simulink model "Marine_LocoMotive_UAV"  (R2018a)
settings: Solver=ode4  StartTime=0.0  StopTime=60  FixedStep=T  RelTol=1e-3
values from neighbouring files (symbols this model uses):
  a_11 = 0.05*m_b    (= 0.625)    [Marine_LocoMotive_UAV_parameters.m]
  a_33 = m_b    (= 12.5)    [Marine_LocoMotive_UAV_parameters.m]
  A_w = 1*1.5/2    (= 0.75)    [Marine_LocoMotive_UAV_parameters.m]
  A_w2 = 1*0.27/2    (= 0.135)    [Marine_LocoMotive_UAV_parameters.m]
  alpha_bar = pi/4    (= 0.785398163397)    [Marine_LocoMotive_UAV_parameters.m]
  Am = sysd.denominator{1}    [Marine_LocoMotive_UAV_parameters.m]
  Am1_LPF = sysd.denominator{1}    [Marine_LocoMotive_UAV_parameters.m]
  Am2_LPF = sysd.denominator{1}    [Marine_LocoMotive_UAV_parameters.m]
  AmAlpha_LPF = sysd.denominator{1}    [Marine_LocoMotive_UAV_parameters.m]
  AmV_LPF = sysd.denominator{1}    [Marine_LocoMotive_UAV_parameters.m]
  AmZ_LPF = sysd.denominator{1}    [Marine_LocoMotive_UAV_parameters.m]
  b_11 = 0    [Marine_LocoMotive_UAV_parameters.m]
  b_33 = 2*m_b*omega_h    (= 27.5578302946)    [Marine_LocoMotive_UAV_parameters.m]
  Bm = sysd.numerator{1}    [Marine_LocoMotive_UAV_parameters.m]
  Bm1_LPF = sysd.numerator{1}    [Marine_LocoMotive_UAV_parameters.m]
  Bm2_LPF = sysd.numerator{1}    [Marine_LocoMotive_UAV_parameters.m]
  BmAlpha_LPF = sysd.numerator{1}    [Marine_LocoMotive_UAV_parameters.m]
  BmV_LPF = sysd.numerator{1}    [Marine_LocoMotive_UAV_parameters.m]
  BmZ_LPF = sysd.numerator{1}    [Marine_LocoMotive_UAV_parameters.m]
  C_S = [5;9]*10^-3    [Marine_LocoMotive_UAV_parameters.m]
  D_x = b_11 + D_s(1)    [Marine_LocoMotive_UAV_parameters.m]
  D_z = b_33 + D_s(2)    [Marine_LocoMotive_UAV_parameters.m]
  dc_M_p = 6.7    [Marine_LocoMotive_UAV_parameters.m]
  Delta_h = (A_im/A_b-0.5)*h_b    (= -0.0625)    [Marine_LocoMotive_UAV_parameters.m]
  epsilon_1 = 5    [Marine_LocoMotive_UAV_parameters.m]
  epsilon_w = 0    [Marine_LocoMotive_UAV_parameters.m]
  epsilon_w2 = pi    (= 3.14159265359)    [Marine_LocoMotive_UAV_parameters.m]
  g = 9.81    [Marine_LocoMotive_UAV_parameters.m]
  gamma_d_p = 2*0.3/0.03*2*0.2*12/4    (= 24)    [Marine_LocoMotive_UAV_parameters.m]
  H = 10    [Marine_LocoMotive_UAV_parameters.m]
  h_b = 0.25    [Marine_LocoMotive_UAV_parameters.m]
  J_a = m_u*Lc_0^2 + (m_u*(Lc_0/2)^2+m_u*Lc_0/12)    (= 111.3)    [Marine_LocoMotive_UAV_parameters.m]
  J_b = m_b*h_b*l_b/12    (= 0.208333333333)    [Marine_LocoMotive_UAV_parameters.m]
  J_u = 0.03    [Marine_LocoMotive_UAV_parameters.m]
  K = 20    [Marine_LocoMotive_UAV_parameters.m]
  k3 = 4.5    [Marine_LocoMotive_UAV_parameters.m]
  k4 = 2    [Marine_LocoMotive_UAV_parameters.m]
  k_w = omega_w^2/g    (= 0.123862835563)    [Marine_LocoMotive_UAV_parameters.m]
  k_w2 = omega_w2^2/g    (= 0.447144836384)    [Marine_LocoMotive_UAV_parameters.m]
  kd_a = 7    [Marine_LocoMotive_UAV_parameters.m]
  kd_t = 6    [Marine_LocoMotive_UAV_parameters.m]
  kd_T = 0.3    [Marine_LocoMotive_UAV_parameters.m]
  kd_x = 5    [Marine_LocoMotive_UAV_parameters.m]
  kd_z = 2    [Marine_LocoMotive_UAV_parameters.m]
  ki_a = 2    [Marine_LocoMotive_UAV_parameters.m]
  ki_T = 0.8    [Marine_LocoMotive_UAV_parameters.m]
  ki_x = 1.2    [Marine_LocoMotive_UAV_parameters.m]
  ki_z = 1    [Marine_LocoMotive_UAV_parameters.m]
  kp_a = 7    [Marine_LocoMotive_UAV_parameters.m]
  kp_t = 10    [Marine_LocoMotive_UAV_parameters.m]
  kp_T = 5    [Marine_LocoMotive_UAV_parameters.m]
  kp_x = 7    [Marine_LocoMotive_UAV_parameters.m]
  kp_z = 3    [Marine_LocoMotive_UAV_parameters.m]
  L = 0.2    [Marine_LocoMotive_UAV_parameters.m]
  l_b = 0.8    [Marine_LocoMotive_UAV_parameters.m]
  Lc_0 = 7    [Marine_LocoMotive_UAV_parameters.m]
  LIMIT_CMD_PITCH = 45*pi/180    (= 0.785398163397)    [Marine_LocoMotive_UAV_parameters.m]
  LIMIT_uCMD_HEIGHT = 3.5*K    (= 70)    [Marine_LocoMotive_UAV_parameters.m]
  M_a = m_u*Lc_0 + m_c*Lc_0    (= 16.1)    [Marine_LocoMotive_UAV_parameters.m]
  m_b = rho_w*Vol_b/4    (= 12.5)    [Marine_LocoMotive_UAV_parameters.m]
  m_c = 0.5    [Marine_LocoMotive_UAV_parameters.m]
  m_u = 1.8    [Marine_LocoMotive_UAV_parameters.m]
  nu_w = 1.787*10^-6    (= 1.787e-06)    [Marine_LocoMotive_UAV_parameters.m]
  omega_w = 2*pi/T_w    (= 1.10231321179)    [Marine_LocoMotive_UAV_parameters.m]
  omega_w2 = 2*pi/T_w2    (= 2.09439510239)    [Marine_LocoMotive_UAV_parameters.m]
  rho_w = 1000    [Marine_LocoMotive_UAV_parameters.m]
  T = 1/100    (= 0.01)    [Marine_LocoMotive_UAV_parameters.m]
  Theta0 = atan2(V_bar*D_x*cos(alpha_bar_0),V_bar*D_x*sin(alpha_bar_0)+m_u*g*cos(alpha_bar_0))    [Marine_LocoMotive_UAV_parameters.m]
  u_s = w_dir*A_w^2*omega_w*k_w*exp(2*k_w*(-Delta_h/2))    [Marine_LocoMotive_UAV_parameters.m]
  u_s2 = w_dir2*A_w2^2*omega_w2*k_w2*exp(2*k_w2*(-Delta_h/2))    [Marine_LocoMotive_UAV_parameters.m]
  u_t = 0*0.2*1    (= 0)    [Marine_LocoMotive_UAV_parameters.m]
  u_w = 0*0.2    (= 0)    [Marine_LocoMotive_UAV_parameters.m]
  V0_b = [u_t+u_w+u_s+u_s2+v_x_w, v_z_w]    [Marine_LocoMotive_UAV_parameters.m]
  V_bar = 5    [Marine_LocoMotive_UAV_parameters.m]
  Vol_b = A_b*l_b    (= 0.05)    [Marine_LocoMotive_UAV_parameters.m]
  w_dir = 1    [Marine_LocoMotive_UAV_parameters.m]
  w_dir2 = 1    [Marine_LocoMotive_UAV_parameters.m]
  X0_b = [0,H+Zeta_0-Delta_h]    [Marine_LocoMotive_UAV_parameters.m]
  zu_bar = X0_b(2) + Lc_0*sin(alpha_bar_0)    [Marine_LocoMotive_UAV_parameters.m]
undefined symbols (not defined in the file or in its folder): DiscIntNeverNeededParam, k_Da, k_Pa, R_b, Zg
libraries: simulink x30, simulink_extras x3
(part 2 of 3)

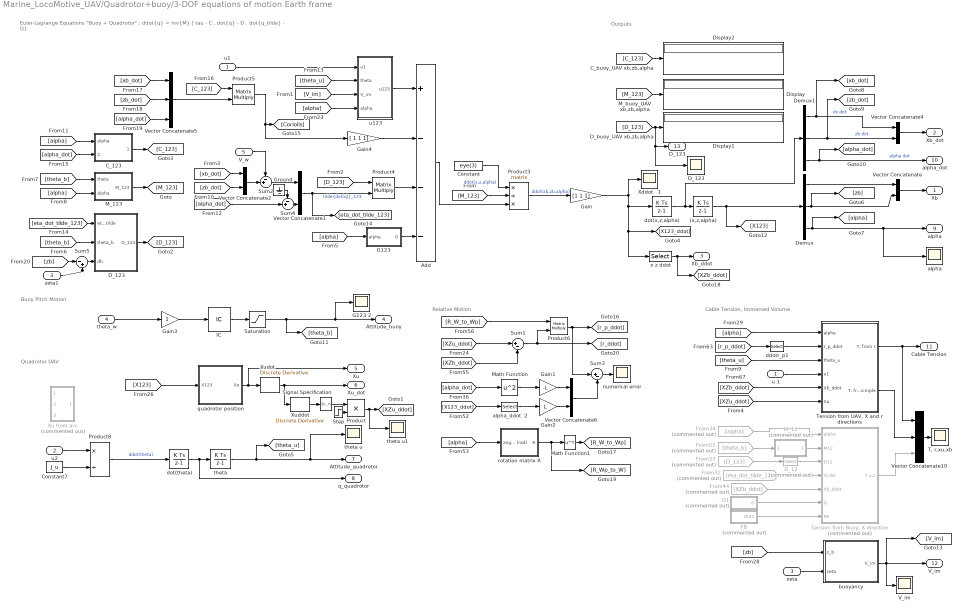
== system Marine_LocoMotive_UAV/Quadrotor+buoy/3-DOF equations of motion Earth frame ==
  note: Relative Motion
  note: Outputs
  note: Buoy Pitch Motion
  note: Cable Tension, Immersed Volume
  note: Quadrotor UAV
  note: Euler-Lagrange Equations "Buoy + Quadrotor" : ddot{q} = inv{M} [ tau - C . dot{q} - D . dot{q_tilde} - G]
  u1 : Inport
  u2 : Inport  Port=2
  zeta : Inport  Port=3
  theta_w : Inport  Port=4
  V_w : Inport  Port=5
  (x,z,alpha) : DiscreteIntegrator  InitialCondition=[pos_b_ini alpha_0]  SampleTime=-1  ICPrevOutput=DiscIntNeverNeededParam  ICPrevScaledInput=DiscIntNeverNeededParam
  Add : Sum  Inputs=+---
  C_123 : Subsystem
  Constant : Constant  Value=eye(3)
  Constant7 : Constant  Value=J_u
  D_12 : Selector  Commented=on  NumberOfDimensions=2  InputPortWidth=3  IndexOptions=Starting index (dialog),Starting index (dialog)  Indices=1,1  OutputSizes=2,2
  D_123 : Subsystem
  "D_123   " : Scope
  Demux : Demux  Outputs=3
  Demux1 : Demux  Outputs=3
  Display : Display
  Display1 : Display
  Display2 : Display
  FB : Subsystem  Commented=on
  From32 : From  Commented=on  GotoTag=eta_dot_tilde_12
  From34 : From  Commented=on  GotoTag=alpha
  From37 : From  Commented=on  GotoTag=D_123
  From44 : From  Commented=on  GotoTag=XZb_ddot
  From51 : From  Commented=on  GotoTag=theta_b
  G1 : Subsystem  Commented=on
  G123 : Subsystem
  G123 2 : Scope
  Gain : Gain  Gain=[1 1 1]
  Gain1 : Gain  Gain=-L
  Gain2 : Gain  Gain=L
  Gain3 : Gain
  Gain4 : Gain  Gain=[ 1 1 1]
  Ground : Ground
  IC : InitialCondition  Value=0
  M_12 : Subsystem  Commented=on
  M_123 : Subsystem
  Math Function : Math  Operator=square  SaturateOnIntegerOverflow=on
  Math Function1 : Math  Operator=transpose  SaturateOnIntegerOverflow=on
  Product : Product
  Product3 : Product  Inputs=*/*  Multiplication=Matrix(*)  SaturateOnIntegerOverflow=on  InputSameDT=on  OutDataTypeStr=Inherit: Same as first input
  Product4 : Product  Inputs=**  Multiplication=Matrix(*)  SaturateOnIntegerOverflow=on  InputSameDT=on  OutDataTypeStr=Inherit: Same as first input
  Product5 : Product  Inputs=**  Multiplication=Matrix(*)  SaturateOnIntegerOverflow=on  InputSameDT=on  OutDataTypeStr=Inherit: Same as first input
  Product6 : Product  Multiplication=Matrix(*)
  Product8 : Product  Inputs=*/  SaturateOnIntegerOverflow=on  InputSameDT=on  OutDataTypeStr=Inherit: Same as first input
  Saturation : Saturate  UpperLimit=0.15  LowerLimit=-0.15
  Signal Specification : SignalSpecification  Dimensions=2
  Step : Step  Time=2*T  SampleTime=0
  Sum1 : Sum  Inputs=|+-
  Sum2 : Sum  Inputs=-+|  SaturateOnIntegerOverflow=on
  Sum3 : Sum  Inputs=|+-
  Sum4 : Sum  Inputs=-+|  SaturateOnIntegerOverflow=on
  Sum5 : Sum  Inputs=|-+  SaturateOnIntegerOverflow=on
  "T, r,xu,xb" : Scope
  "Tension from Buoy, X direction" : Subsystem  Commented=on
  "Tension from UAV, X and r directions" : Subsystem
  "V_im " : Scope
  Vector Concatenate{,1..2,4,6} (5 alike) : Concatenate
  Vector Concatenate10 : Concatenate  NumInputs=3
  Vector Concatenate5 : Concatenate  NumInputs=3
  Xddot   1 : Scope
  Xu from acc : Subsystem  Commented=on
  Xuddot : simulink/Discrete/Discrete Derivative  gainval=1.0  ICPrevScaledInput=[v_b_ini]/T  OutMin=[]  OutMax=[]  OutDataType=fixdt(1, 16)  OutScaling=2^-10  DoSatur=off
  Xudot : simulink/Discrete/Discrete Derivative  gainval=1.0  ICPrevScaledInput=(pos_b_ini+Lc_0*[cos(alpha_0) sin(alpha_0)])/T  OutMin=[]  OutMax=[]  OutDataType=fixdt(1, 16)  OutScaling=2^-10  DoSatur=off
  "alpha  " : Scope
  alpha_ddot  2 : Selector  InputPortWidth=3  IndexOptions=Index vector (dialog)  Indices=3  OutputSizes=2
  buoyancy : Subsystem
  ddotr_p1 : Selector  InputPortWidth=2  IndexOptions=Index vector (dialog)  Indices=1  OutputSizes=2
  dot(theta) : DiscreteIntegrator  gainval=1  InitialCondition=q_b_ini  SampleTime=-1  ICPrevOutput=DiscIntNeverNeededParam  ICPrevScaledInput=DiscIntNeverNeededParam
  dot(x,z,alpha) : DiscreteIntegrator  InitialCondition=[v_b_ini 0]  SampleTime=-1  ICPrevOutput=DiscIntNeverNeededParam  ICPrevScaledInput=DiscIntNeverNeededParam
  numerical error : Scope
  quadrotor position : Subsystem
  "rotation matrix R " : Subsystem
  theta : DiscreteIntegrator  InitialCondition=theta_q_ini  SampleTime=-1  StateName=theta  ICPrevOutput=DiscIntNeverNeededParam  ICPrevScaledInput=DiscIntNeverNeededParam
  theta u : Scope
  theta u1 : Scope
  u 1 : InportShadow
  u123 : Subsystem
  x z ddot : Selector  InputPortWidth=3  IndexOptions=Index vector (dialog)  Indices=[1 2]  OutputSizes=1
  zeta1 : InportShadow  Port=3
  Xb : Outport  Unit=m  InitialOutput=0
  Xb_dot : Outport  Port=2  Unit=m  InitialOutput=0
  Xb_ddot : Outport  Port=3  Unit=m  InitialOutput=0
  Attitude_buoy : Outport  Port=4  Unit=rad/s^2  InitialOutput=0
  Xu : Outport  Port=5  Unit=m  InitialOutput=0
  Xu_dot : Outport  Port=6  Unit=m/s  InitialOutput=0
  Attitude_quadrotor : Outport  Port=7  Unit=rad  InitialOutput=0
  q_quadrotor : Outport  Port=8  Unit=rad/s  InitialOutput=0
  alpha : Outport  Port=9  Unit=m  InitialOutput=0
  alpha_dot : Outport  Port=10  Unit=m  InitialOutput=0
  Cable Tension : Outport  Port=11  Unit=rad/s^2  InitialOutput=0
  V_im : Outport  Port=12  Unit=m  InitialOutput=0
  "D_123 " : Outport  Port=13  Unit=m  InitialOutput=0
  wires:
  Vector Concatenate/1 -> Xb/1
  dot(x,z,alpha)/1 -> Demux1/1, (x,z,alpha)/1
  u123/1(u123) -> Add/1
  Product4/1 -> Add/3
  [D_123] -> Product4/1
  Vector Concatenate1/1 -> [eta_dot_tilde_123], Product4/2  "tilde{dot(q)}_123"
  G123/1(G) -> Add/4
  Demux/3 -> "alpha  "/1, alpha/1, [alpha]
  [theta_b] -> D_123/2(theta_b)
  D_123/1(D_123) -> [D_123]
  [theta_b] -> M_123/1(theta)
  [alpha] -> M_123/2(alpha)
  Demux1/2 -> [zb_dot], Vector Concatenate4/2  "zb dot"
  Demux1/1 -> [xb_dot], Vector Concatenate4/1  "xb dot"
  [xb_dot] -> Vector Concatenate2/1
  [zb_dot] -> Vector Concatenate2/2
  Vector Concatenate2/1 -> Sum2/2
  V_w/1 -> Sum2/1
  Sum2/1 -> Vector Concatenate1/1
  Sum4/1 -> Vector Concatenate1/2
  theta_w/1 -> Gain3/1
  dot(theta)/1 -> q_quadrotor/1, theta/1
  theta/1 -> [theta_u], theta u/1, Attitude_quadrotor/1
  Constant7/1 -> Product8/2
  u2/1 -> Product8/1
  u1/1 -> u123/1(u1)
  [theta_u] -> u123/2(theta)
  [V_im] -> u123/3(V_im)
  [alpha] -> G123/1(alpha)
  Demux/1 -> Vector Concatenate/1
  Demux/2 -> [zb], Vector Concatenate/2
  Vector Concatenate4/1 -> Xb_dot/1
  M_123/1(M_123) -> [M_123]
  Product8/1 -> dot(theta)/1  "ddot(theta)"
  [M_123] -> Product3/2
  Constant/1 -> Product3/1  "ddot(x,z,alpha)"
  Product3/1 -> Gain/1  "ddot(xb,zb,alpha)"
  IC/1 -> Saturation/1
  Xuddot/1 -> Signal Specification/1
  [alpha] -> C_123/1("alpha ")
  [alpha_dot] -> C_123/2(alpha_dot)
  C_123/1(C_123) -> [C_123]
  Vector Concatenate5/1 -> Product5/2
  [xb_dot] -> Vector Concatenate5/1
  [zb_dot] -> Vector Concatenate5/2
  [alpha_dot] -> Vector Concatenate5/3
  [C_123] -> Product5/1
  Product5/1 -> [Coriolis], Gain4/1
  Demux1/3 -> alpha_dot/1, [alpha_dot]  "alpha dot"
  Gain/1 -> Xddot   1/1, x z ddot/1, [X123_ddot], dot(x,z,alpha)/1
  [alpha] -> u123/4(alpha)
  [r_p_ddot] -> ddotr_p1/1
  [alpha] -> "Tension from UAV, X and r directions"/1(alpha)
  [theta_u] -> "Tension from UAV, X and r directions"/3(theta_u)
  u 1/1 -> "Tension from UAV, X and r directions"/4(u1)
  [D_123] -> "D_123 "/1, "D_123   "/1, Display1/1
  [M_123] -> Display/1
  [C_123] -> Display2/1
  (x,z,alpha)/1 -> [X123], Demux/1
  [X123] -> quadrotor position/1(X123)
  [zb] -> buoyancy/1(z_b)
  zeta/1 -> buoyancy/2(zeta)
  From34/1 -> "Tension from Buoy, X direction"/1(alpha)
  D_12/1 -> "Tension from Buoy, X direction"/3(D12)
  buoyancy/1(V_im) -> "V_im "/1, V_im/1, [V_im]
  M_12/1(M_12) -> "Tension from Buoy, X direction"/2(M12)
  From37/1 -> D_12/1
  From44/1 -> "Tension from Buoy, X direction"/5(Xb_ddot)
  From32/1 -> "Tension from Buoy, X direction"/4(Vr,Wr)
  Xudot/1 -> Xu_dot/1, Xuddot/1
  Step/1 -> Product/2
  Signal Specification/1 -> Product/1
  Product/1 -> theta u1/1, [XZu_ddot]
  [XZb_ddot] -> "Tension from UAV, X and r directions"/5(Xb_ddot)
  G1/1(G) -> "Tension from Buoy, X direction"/6(G)
  From51/1 -> M_12/1(theta)
  x z ddot/1 -> [XZb_ddot], Xb_ddot/1
  quadrotor position/1(Xu) -> Xu/1, Xudot/1
  "Tension from UAV, X and r directions"/1("T, from r") -> Vector Concatenate10/1, Cable Tension/1
  ddotr_p1/1 -> "Tension from UAV, X and r directions"/2(r_p_ddot)
  [XZu_ddot] -> "Tension from UAV, X and r directions"/6(Xu)
  FB/1(Out1) -> "Tension from Buoy, X direction"/7(FB)
  Vector Concatenate10/1 -> "T, r,xu,xb"/1
  "Tension from UAV, X and r directions"/2("T, from x simple") -> Vector Concatenate10/2
  "Tension from Buoy, X direction"/1(T x,z) -> Vector Concatenate10/3
  Gain2/1 -> Vector Concatenate6/2
  [R_W_to_Wp] -> Product6/1
  [X123_ddot] -> alpha_ddot  2/1
  Vector Concatenate6/1 -> Sum3/2
  "rotation matrix R "/1(R) -> [R_Wp_to_W], Math Function1/1
  Product6/1 -> Sum3/1, [r_p_ddot]
  Gain1/1 -> Vector Concatenate6/1
  Math Function/1 -> Gain1/1
  Sum1/1 -> Product6/2, [r_ddot]
  [XZu_ddot] -> Sum1/1
  alpha_ddot  2/1 -> Gain2/1
  Math Function1/1 -> [R_W_to_Wp]
  Sum3/1 -> numerical error/1
  [XZb_ddot] -> Sum1/2
  [alpha] -> "rotation matrix R "/1(angle (rad))
  [alpha_dot] -> Math Function/1
  Saturation/1 -> G123 2/1, Attitude_buoy/1, [theta_b]
  Add/1 -> Product3/3
  Gain3/1 -> IC/1
  Gain4/1 -> Add/2
  [alpha_dot] -> Sum4/2
  Ground/1 -> Sum4/1
  [eta_dot_tilde_123] -> D_123/1(eta_dot_tilde)
  Sum5/1 -> D_123/3(dh)
  [zb] -> Sum5/1
  zeta1/1 -> Sum5/2

== system Marine_LocoMotive_UAV/Reference Governer/Alpha_bar ==
  zb : Inport
  zq_bar : Inport  Port=2
  Constant1 : Constant  Value=Lc_0^2
  Product : Product
  Sqrt : Sqrt  SaturateOnIntegerOverflow=on
  Sum : Sum  Inputs=|+-
  Sum1 : Sum  Inputs=|+-
  "alpha_bar " : Trigonometry  Operator=atan2
  alpha_bar : Outport
  wires:
  "alpha_bar "/1 -> alpha_bar/1
  Sqrt/1 -> "alpha_bar "/2
  Sum/1 -> "alpha_bar "/1, Product/1, Product/2
  Sum1/1 -> Sqrt/1
  zb/1 -> Sum/2
  Constant1/1 -> Sum1/1
  Product/1 -> Sum1/2
  zq_bar/1 -> Sum/1

== system Marine_LocoMotive_UAV/Reference Governer/Subsystem ==
  Vr_bar : Inport
  Dh_bar : Inport  Port=2
  C_S : Inport  Port=3
  Abs : Abs
  Bias2 : Bias  Bias=b_11
  Constant : Constant  Value=D_x
  Constant2 : Constant  Value=0.5*rho_w
  "D11  " : Scope
  Dx : Scope
  Gain1 : Gain  Gain=2*l_b
  Manual Switch : ManualSwitch  CurrentSetting=0
  Product6 : Product  Inputs=4
  Sum5 : Sum  Inputs=|++  SaturateOnIntegerOverflow=on
  bottom plan : Constant  Value=l_b*h_b
  D11 : Outport
  wires:
  Constant2/1 -> Product6/3
  Abs/1 -> Product6/1
  Gain1/1 -> Sum5/1
  Sum5/1 -> Product6/2  "Aw"
  Dh_bar/1 -> Gain1/1
  bottom plan/1 -> Sum5/2
  C_S/1 -> Product6/4
  Vr_bar/1 -> Abs/1
  Product6/1 -> Bias2/1
  Bias2/1 -> "D11  "/1, Manual Switch/2
  Manual Switch/1 -> D11/1
  Constant/1 -> Manual Switch/1, Dx/1

== system Marine_LocoMotive_UAV/Reference Governer/Subsystem1 ==
  Vol_im_bar : Inport
  Constant : Constant  Value=Vol_b
  Product : Product
  Vol im ratio : Product  Inputs=*/
  height : Constant  Value=h_b
  Dh_bar : Outport
  wires:
  Vol_im_bar/1 -> Vol im ratio/1
  Vol im ratio/1 -> Product/2
  height/1 -> Product/1
  Product/1 -> Dh_bar/1
  Constant/1 -> Vol im ratio/2

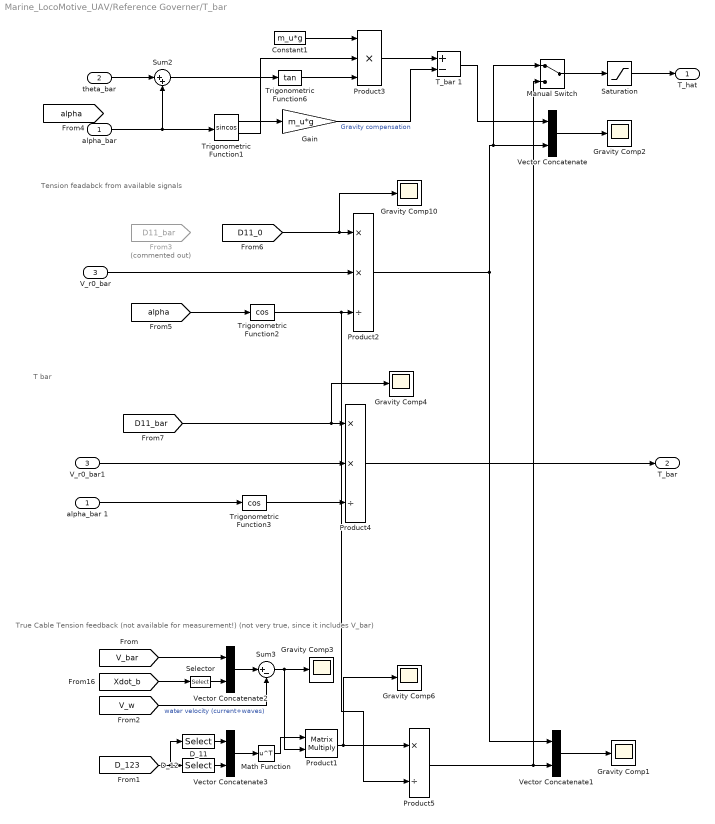
== system Marine_LocoMotive_UAV/Reference Governer/T_bar  ==
  note: Tension feadabck from available signals
  note: True Cable Tension feedback (not available for measurement!) (not very true, since it includes V_bar)
  note: T bar
  "alpha_bar " : Inport
  theta_bar : Inport  Port=2
  V_r0_bar : Inport  Port=3
  Constant1 : Constant  Value=m_u*g
  D_11 : Selector  NumberOfDimensions=2  InputPortWidth=2  IndexOptions=Index vector (dialog),Index vector (dialog)  Indices=1,1  OutputSizes=1,1
  D_12 : Selector  NumberOfDimensions=2  InputPortWidth=2  IndexOptions=Index vector (dialog),Index vector (dialog)  Indices=1,2  OutputSizes=1,1
  From3 : From  Commented=on  GotoTag=D11_bar  TagVisibility=global
  Gain : Gain  Gain=m_u*g
  Gravity Comp{1..4,6,10} (6 alike) : Scope
  Manual Switch : ManualSwitch
  Math Function : Math  Operator=transpose  SaturateOnIntegerOverflow=on
  Product1 : Product  Multiplication=Matrix(*)
  Product2 : Product  Inputs=**/
  Product3 : Product  Inputs=***
  Product4 : Product  Inputs=**/
  Product5 : Product  Inputs=*/
  Saturation : Saturate  UpperLimit=inf  LowerLimit=epsilon_1
  Selector : Selector  InputPortWidth=2  IndexOptions=Index vector (dialog)  Indices=2  OutputSizes=1
  Sum2 : Sum  Inputs=|++
  Sum3 : Sum  Inputs=|+-
  T_bar 1 : Sum  Inputs=+-
  Trigonometric Function1 : Trigonometry  Operator=sincos
  Trigonometric Function2 : Trigonometry  Operator=cos
  Trigonometric Function3 : Trigonometry  Operator=cos
  Trigonometric Function6 : Trigonometry  Operator=tan
  V_r0_bar1 : InportShadow  Port=3
  Vector Concatenate{,1..3} (4 alike) : Concatenate
  alpha_bar 1 : InportShadow
  T_hat : Outport
  T_bar : Outport  Port=2
  wires:
  "alpha_bar "/1 -> Sum2/2, Trigonometric Function1/1
  Trigonometric Function1/1 -> Gain/1
  Gain/1 -> T_bar 1/2  "Gravity compensation"
  theta_bar/1 -> Sum2/1
  Sum2/1 -> Trigonometric Function6/1
  Vector Concatenate1/1 -> Gravity Comp1/1
  [D11_0] -> Gravity Comp10/1, Product2/1
  Product2/1 -> Manual Switch/1, Vector Concatenate/2, Vector Concatenate1/1
  Vector Concatenate/1 -> Gravity Comp2/1
  Saturation/1 -> T_hat/1
  Constant1/1 -> Product3/1
  Trigonometric Function1/2 -> Product3/2
  Trigonometric Function6/1 -> Product3/3
  Product3/1 -> T_bar 1/1
  [D_123] -> D_11/1, D_12/1
  D_11/1 -> Vector Concatenate3/1
  [Xdot_b] -> Selector/1
  Sum3/1 -> Product1/2, Gravity Comp3/1
  Vector Concatenate2/1 -> Sum3/1
  [V_w] -> Sum3/2  "water velocity (current+waves)"
  Product1/1 -> Gravity Comp6/1, Product5/1
  Product5/1 -> Manual Switch/2, Vector Concatenate1/2
  Manual Switch/1 -> Saturation/1
  T_bar 1/1 -> Vector Concatenate/1
  V_r0_bar/1 -> Product2/2
  [alpha] -> Trigonometric Function2/1
  Trigonometric Function2/1 -> Product5/2, Product2/3
  [V_bar] -> Vector Concatenate2/1
  Selector/1 -> Vector Concatenate2/2
  D_12/1 -> Vector Concatenate3/2
  Vector Concatenate3/1 -> Math Function/1
  Math Function/1 -> Product1/1
  alpha_bar 1/1 -> Trigonometric Function3/1
  V_r0_bar1/1 -> Product4/2
  [D11_bar] -> Product4/1, Gravity Comp4/1
  Trigonometric Function3/1 -> Product4/3
  Product4/1 -> T_bar/1

== system Marine_LocoMotive_UAV/Reference Governer/Theta_bar  ==
  "alpha_bar " : Inport
  V_r0_bar : Inport  Port=2
  D11_bar : Inport  Port=3
  Add : Sum
  D_11 : Selector  NumberOfDimensions=2  InputPortWidth=2  IndexOptions=Index vector (dialog),Index vector (dialog)  Indices=1,1  OutputSizes=1,1
  Gain : Gain  Gain=m_u*g
  Mux : Mux  Inputs=2
  Product1 : Product
  Product2 : Product  Inputs=**
  Product3 : Product
  Scope : Scope
  Trigonometric Function3 : Trigonometry  Operator=sincos
  "theta_bar " : Trigonometry  Operator=atan2
  theta_bar : Outport
  wires:
  "theta_bar "/1 -> theta_bar/1
  "alpha_bar "/1 -> Trigonometric Function3/1
  Product1/1 -> "theta_bar "/1  "dy"
  Add/1 -> "theta_bar "/2  "dx"
  Product2/1 -> Add/1
  Trigonometric Function3/1 -> Product2/1
  Trigonometric Function3/2 -> Product1/2, Gain/1
  Gain/1 -> Add/2
  [D_123] -> D_11/1
  V_r0_bar/1 -> Product3/2
  Product3/1 -> Product2/2, Product1/1
  D11_bar/1 -> Mux/2, Product3/1
  Mux/1 -> Scope/1
  D_11/1 -> Mux/1

== system Marine_LocoMotive_UAV/Reference Governer/damping estimates ==
  V_bar : Inport
  C_S_bar : Inport  Port=2
  Abs1 : Abs
  Bias : Bias  Bias=h_b/2
  Bias2 : Bias  Bias=b_11
  Constant : Constant  Value=D_x
  Constant2 : Constant  Value=0.5*rho_w
  "D11  " : Scope
  Dh @ no tension : Constant  Value=Delta_h
  Dx : Scope
  Dx1 : Scope
  Gain1 : Gain  Gain=2*l_b
  Manual Switch : ManualSwitch  CurrentSetting=0
  Product6 : Product  Inputs=4
  Saturation : Saturate  UpperLimit=h_b  LowerLimit=0
  Sum5 : Sum  Inputs=|++  SaturateOnIntegerOverflow=on
  bottom plan : Constant  Value=l_b*h_b
  D11,0 : Outport
  wires:
  Constant/1 -> Dx/1, Manual Switch/1
  Manual Switch/1 -> D11,0/1
  Bias2/1 -> Manual Switch/2, "D11  "/1
  Product6/1 -> Bias2/1
  C_S_bar/1 -> Product6/4
  bottom plan/1 -> Sum5/2
  Dh @ no tension/1 -> Bias/1
  Sum5/1 -> Dx1/1, Product6/2  "Aw"
  Gain1/1 -> Sum5/1
  V_bar/1 -> Abs1/1
  Constant2/1 -> Product6/3
  Abs1/1 -> Product6/1
  Bias/1 -> Saturation/1
  Saturation/1 -> Gain1/1

== system Marine_LocoMotive_UAV/Reference Governer/mean skin friction coefficient  ==
  V : Inport
  Abs1 : Abs
  C_S Lewis1988 : Fcn  Expr=0.075/(log10(u(1))-2)^2
  Re Reynolds number : Gain  Gain=l_b/nu_w
  Saturation1 : Saturate  UpperLimit=inf  LowerLimit=0.5*10^5
  C_S : Outport
  wires:
  Re Reynolds number/1 -> Saturation1/1
  Abs1/1 -> Re Reynolds number/1
  Saturation1/1 -> C_S Lewis1988/1
  V/1 -> Abs1/1
  C_S Lewis1988/1 -> C_S/1

== system Marine_LocoMotive_UAV/Save to file/mean absolute error ==
  In1 : Inport
  Abs : Abs
  Add : Sum
  Constant : Constant  Value=T
  Delay : Delay  DelayLength=1
  IC : InitialCondition
  Product1 : Product  Inputs=*/
  Product2 : Product  Inputs=*/
  Out1 : Outport
  wires:
  Product2/1 -> IC/1
  Add/1 -> Product1/1, Delay/1
  Delay/1 -> Add/1
  [time] -> Product2/1
  In1/1 -> Abs/1
  Product1/1 -> Out1/1
  Constant/1 -> Product2/2
  IC/1 -> Product1/2
  Abs/1 -> Add/2

== system Marine_LocoMotive_UAV/Scope/Subsystem ==
  In1 : Inport
  In2 : Inport  Port=2
  Product : Product
  Sqrt : Sqrt  SaturateOnIntegerOverflow=on
  Subtract : Sum  Inputs=+-
  Sum of Elements : Sum  Inputs=+
  Out1 : Outport
  wires:
  In1/1 -> Subtract/2
  Product/1 -> Sum of Elements/1
  Subtract/1 -> Product/2, Product/1
  In2/1 -> Subtract/1
  Sqrt/1 -> Out1/1, [r]
  Sum of Elements/1 -> Sqrt/1

== system Marine_LocoMotive_UAV/Scope/absolute mean ==
  u : Inport
  Abs : Abs
  Clock : Clock
  Current velocity : Scope
  Current velocity1 : Scope
  Current velocity2 : Scope
  Discrete-Time Integrator : DiscreteIntegrator  gainval=1  SampleTime=T  ICPrevOutput=DiscIntNeverNeededParam  ICPrevScaledInput=DiscIntNeverNeededParam
  Divide1 : Product  Inputs=*/
  mean : Outport
  wires:
  Discrete-Time Integrator/1 -> Current velocity1/1, Divide1/1
  Abs/1 -> Discrete-Time Integrator/1
  u/1 -> Current velocity/1, Abs/1
  Divide1/1 -> mean/1
  Clock/1 -> Current velocity2/1, Divide1/2

== system Marine_LocoMotive_UAV/Scope/absolute mean1 ==
  u : Inport
  Abs : Abs
  Clock : Clock
  Current velocity : Scope
  Current velocity1 : Scope
  Current velocity2 : Scope
  Discrete-Time Integrator : DiscreteIntegrator  gainval=1  SampleTime=T  ICPrevOutput=DiscIntNeverNeededParam  ICPrevScaledInput=DiscIntNeverNeededParam
  Divide1 : Product  Inputs=*/
  mean : Outport
  wires:
  Clock/1 -> Divide1/2, Current velocity2/1
  Divide1/1 -> mean/1
  u/1 -> Abs/1, Current velocity/1
  Abs/1 -> Discrete-Time Integrator/1
  Discrete-Time Integrator/1 -> Divide1/1, Current velocity1/1

== system Marine_LocoMotive_UAV/Sea/Single Wave ==
  note: Aw.Sin
  time : Inport
  x(t) : Inport  Port=2
  Constant : Constant  Value=epsilon
  Gain : Gain  Gain=omega
  Gain1 : Gain  Gain=k
  Gain2 : Gain  Gain=A
  Gain3 : Gain  Gain=omega*A
  Gain4 : Gain  Gain=omega*A
  Gain5 : Gain  Gain=A*k
  Sum : Sum  Inputs=++-
  Trigonometric Function : Trigonometry  Operator=sincos
  Trigonometric Function1 : Trigonometry  Operator=atan
  direction : Gain  Gain=w_dir
  direction1 : Gain  Gain=w_dir
  direction2 : Gain  Gain=w_dir
  zeta(x,t) : Outport
  theta_w(x,t) : Outport  Port=2
  u(z0,x,t) : Outport  Port=3
  w(z0,x,t) : Outport  Port=4
  wires:
  Gain/1 -> Sum/2
  Gain1/1 -> Sum/3
  x(t)/1 -> Gain1/1
  Trigonometric Function/1 -> Gain3/1, Gain2/1
  Constant/1 -> Sum/1
  time/1 -> direction/1
  direction/1 -> Gain/1
  Gain2/1 -> zeta(x,t)/1  "zeta(x,t)"
  Trigonometric Function/2 -> Gain5/1, Gain4/1
  Sum/1 -> Trigonometric Function/1
  Trigonometric Function1/1 -> theta_w(x,t)/1
  Gain5/1 -> Trigonometric Function1/1
  Gain3/1 -> direction1/1
  Gain4/1 -> direction2/1
  direction1/1 -> u(z0,x,t)/1
  direction2/1 -> w(z0,x,t)/1

== system Marine_LocoMotive_UAV/Sea/Single Wave1 ==
  note: Aw.Sin
  time : Inport
  x(t) : Inport  Port=2
  Constant : Constant  Value=epsilon
  Gain : Gain  Gain=omega
  Gain1 : Gain  Gain=k
  Gain2 : Gain  Gain=A
  Gain3 : Gain  Gain=omega*A
  Gain4 : Gain  Gain=omega*A
  Gain5 : Gain  Gain=A*k
  Sum : Sum  Inputs=++-
  Trigonometric Function : Trigonometry  Operator=sincos
  Trigonometric Function1 : Trigonometry  Operator=atan
  direction : Gain  Gain=w_dir
  direction1 : Gain  Gain=w_dir
  direction2 : Gain  Gain=w_dir
  zeta(x,t) : Outport
  theta_w(x,t) : Outport  Port=2
  u(z0,x,t) : Outport  Port=3
  w(z0,x,t) : Outport  Port=4
  wires:
  direction2/1 -> w(z0,x,t)/1
  direction1/1 -> u(z0,x,t)/1
  Gain4/1 -> direction2/1
  Gain3/1 -> direction1/1
  Gain5/1 -> Trigonometric Function1/1
  Trigonometric Function1/1 -> theta_w(x,t)/1
  Sum/1 -> Trigonometric Function/1
  Trigonometric Function/2 -> Gain4/1, Gain5/1
  Gain2/1 -> zeta(x,t)/1  "zeta(x,t)"
  direction/1 -> Gain/1
  time/1 -> direction/1
  Constant/1 -> Sum/1
  Trigonometric Function/1 -> Gain2/1, Gain3/1
  x(t)/1 -> Gain1/1
  Gain1/1 -> Sum/3
  Gain/1 -> Sum/2

== system Marine_LocoMotive_UAV/Sea/Theta_water surface (two waves) ==
  w1 : Inport
  w2 : Inport  Port=2
  Gain2 : Gain  Gain=1/(omega_w)
  Gain3 : Gain  Gain=k_w
  Gain4 : Gain  Gain=1/(omega_w2)
  Gain5 : Gain  Gain=k_w2
  Sum2 : Sum  Inputs=++|
  direction1 : Gain  Gain=1/w_dir
  direction2 : Gain  Gain=1/w_dir2
  Out1 : Outport
  wires:
  Gain4/1 -> direction2/1
  direction2/1 -> Gain5/1
  Sum2/1 -> Out1/1
  w1/1 -> Gain2/1
  Gain3/1 -> Sum2/1
  Gain5/1 -> Sum2/2
  w2/1 -> Gain4/1
  direction1/1 -> Gain3/1
  Gain2/1 -> direction1/1

== system Marine_LocoMotive_UAV/Sea1/Single Wave ==
  note: Aw.Sin
  time : Inport
  x(t) : Inport  Port=2
  Bias : Bias  Bias=H
  Constant : Constant  Value=epsilon_w
  Gain : Gain  Gain=omega_w
  Gain1 : Gain  Gain=k_w
  Gain2 : Gain  Gain=A_w
  Gain3 : Gain  Gain=A_w*k_w
  Gain5 : Gain  Gain=A_w*k_w
  Gain6 : Gain  Gain=w_dir
  Sum : Sum  Inputs=++-
  Trigonometric Function : Trigonometry  Operator=sincos
  Trigonometric Function1 : Trigonometry  Operator=atan
  zeta(x,t) : Outport
  theta_w(x,t) : Outport  Port=2
  u(z0,x,t) : Outport  Port=3
  w(z0,x,t) : Outport  Port=4
  wires:
  Gain3/1 -> u(z0,x,t)/1
  Gain5/1 -> Trigonometric Function1/1, w(z0,x,t)/1
  Trigonometric Function1/1 -> theta_w(x,t)/1
  Sum/1 -> Trigonometric Function/1
  Trigonometric Function/2 -> Gain5/1  "w(x,t)"
  Bias/1 -> zeta(x,t)/1  "zeta(x,t)"
  Gain6/1 -> Gain/1
  time/1 -> Gain6/1
  Gain2/1 -> Bias/1
  Constant/1 -> Sum/1
  Trigonometric Function/1 -> Gain2/1, Gain3/1
  x(t)/1 -> Gain1/1
  Gain1/1 -> Sum/3
  Gain/1 -> Sum/2

== system Marine_LocoMotive_UAV/UAV control/Coupling ==
  U1 : Inport
  U3 : Inport  Port=2
  Coupling : Subsystem
  sat : Subsystem
  u_1 : Outport
  theta_d : Outport  Port=2
  wires:
  Coupling/1(u1 (N)) -> u_1/1
  Coupling/2(phi_d (rad)) -> sat/1(u)
  U3/1 -> Coupling/2(U3)
  U1/1 -> Coupling/1(U1)
  sat/1(sat(u)) -> theta_d/1

== system Marine_LocoMotive_UAV/UAV control/Coupling  ==
  u_T : Inport
  u_a : Inport  Port=2
  alpha : Inport  Port=3
  Add5 : Sum  Inputs=2
  Bias : Bias  Bias=-pi/2
  Product1 : Product
  Product3 : Product
  Saturation : Saturate  UpperLimit=LIMIT_uCMD_HEIGHT  LowerLimit=m_u*g*0.5
  Scope{,1..5} (6 alike) : Scope
  Sqrt : Sqrt  SaturateOnIntegerOverflow=on
  Subtract : Sum  Inputs=--
  Trigonometric Function1 : Trigonometry  Operator=atan2
  Vector Concatenate : Concatenate
  "sat " : Subsystem
  u1 : Outport
  theta_c : Outport  Port=2
  wires:
  Bias/1 -> Scope2/1, Subtract/1
  Product1/1 -> Add5/1, Scope/1
  Sqrt/1 -> Saturation/1
  Subtract/1 -> "sat "/1(u)
  Trigonometric Function1/1 -> Scope4/1, Subtract/2
  Product3/1 -> Scope1/1, Add5/2
  Add5/1 -> Sqrt/1
  alpha/1 -> Bias/1
  Saturation/1 -> u1/1
  "sat "/1(sat(u)) -> Scope3/1, theta_c/1
  u_a/1 -> Vector Concatenate/1, Trigonometric Function1/1, Product3/1, Product3/2
  u_T/1 -> Product1/2, Product1/1, Vector Concatenate/2, Trigonometric Function1/2
  Vector Concatenate/1 -> Scope5/1

== system Marine_LocoMotive_UAV/UAV control/Subsystem ==
  In1 : Inport
  In2 : Inport  Port=2
  In3 : Inport  Port=3
  In4 : Inport  Port=4
  Add1 : Sum
  Gain1 : Gain  Gain=k_Da
  Gain2 : Gain  Gain=k_Pa
  Sum5 : Sum  Inputs=|+-
  Sum6 : Sum  Inputs=|+-
  Out1 : Outport
  wires:
  Add1/1 -> Out1/1
  Sum5/1 -> Gain2/1
  In4/1 -> Sum6/2
  Gain2/1 -> Add1/1
  Gain1/1 -> Add1/2
  In2/1 -> Sum5/2
  Sum6/1 -> Gain1/1
  In1/1 -> Sum5/1
  In3/1 -> Sum6/1

== system Marine_LocoMotive_UAV/UAV control/V control ==
  V_bar : Inport
  V : Inport  Port=2
  Discrete Derivative1 : simulink/Discrete/Discrete Derivative  gainval=1.0  ICPrevScaledInput=0.0  OutMin=[]  OutMax=[]  OutDataType=fixdt(1, 16)  OutScaling=2^-10  DoSatur=off
  Discrete Derivative6 : simulink/Discrete/Discrete Derivative  gainval=1.0  ICPrevScaledInput=0.0  OutMin=[]  OutMax=[]  OutDataType=fixdt(1, 16)  OutScaling=2^-10  DoSatur=off
  Discrete-Time Integrator : DiscreteIntegrator  SampleTime=-1  LimitOutput=on  UpperSaturationLimit=300  LowerSaturationLimit=-200  ICPrevOutput=DiscIntNeverNeededParam  ICPrevScaledInput=DiscIntNeverNeededParam
  Gain : Gain  Gain=ki_x
  IC : InitialCondition  Value=0
  IC1 : InitialCondition  Value=0
  IC2 : InitialCondition  Value=0
  K1 : Gain  Gain=kp_x
  K2 : Gain  Gain=kd_x
  K3 : Gain
  K4 : Gain
  Mux : Mux  Inputs=2
  Mux1 : Mux  Inputs=2
  Product : Product
  Saturation1 : Saturate  UpperLimit=50  LowerLimit=-20
  Scope{1..6} (6 alike) : Scope
  Step : Step  Time=3*T  SampleTime=0
  Sum : Sum  Inputs=|+-
  Sum1 : Sum  Inputs=|+-
  Sum4 : Sum  Inputs=---
  U1 (m/s^2) : Outport
  wires:
  Sum1/1 -> Product/1  "ev"
  Sum/1 -> Discrete-Time Integrator/1, K1/1  "ex"
  V_bar/1 -> Mux/2, Sum/2, Discrete Derivative6/1
  Sum4/1 -> Saturation1/1
  K1/1 -> K4/1
  K2/1 -> K3/1
  Discrete-Time Integrator/1 -> Gain/1
  Gain/1 -> Scope3/1, Sum4/3
  Saturation1/1 -> Scope4/1, U1 (m/s^2)/1
  Mux/1 -> Scope1/1
  Discrete Derivative1/1 -> IC1/1
  Mux1/1 -> Scope2/1
  Discrete Derivative6/1 -> IC2/1
  IC/1 -> Discrete Derivative1/1, Mux/1, Sum/1
  V/1 -> IC/1
  IC1/1 -> Sum1/1, Mux1/1
  IC2/1 -> Mux1/2, Sum1/2
  K3/1 -> Scope5/1, Sum4/2
  K4/1 -> Scope6/1, Sum4/1
  Product/1 -> K2/1
  Step/1 -> Product/2

== system Marine_LocoMotive_UAV/UAV control/Z controller ==
  z_bar : Inport
  z_u : Inport  Port=2
  Constant : Constant  Value=g
  Discrete Derivative1 : simulink/Discrete/Discrete Derivative  gainval=1.0  ICPrevScaledInput=0.0  OutMin=[]  OutMax=[]  OutDataType=fixdt(1, 16)  OutScaling=2^-10  DoSatur=off
  Discrete Derivative6 : simulink/Discrete/Discrete Derivative  gainval=1.0  ICPrevScaledInput=0.0  OutMin=[]  OutMax=[]  OutDataType=fixdt(1, 16)  OutScaling=2^-10  DoSatur=off
  Discrete-Time Integrator : DiscreteIntegrator  SampleTime=-1  LimitOutput=on  UpperSaturationLimit=100  LowerSaturationLimit=-100  ICPrevOutput=DiscIntNeverNeededParam  ICPrevScaledInput=DiscIntNeverNeededParam
  Divide : Product  Inputs=*/
  Gain : Gain  Gain=ki_z
  IC : InitialCondition  Value=0
  IC1 : InitialCondition  Value=0
  K1 : Gain  Gain=kp_z
  K2 : Gain  Gain=kd_z
  K3 : Gain
  Mux : Mux  Inputs=2
  Mux1 : Mux  Inputs=2
  Saturation1 : Saturate  UpperLimit=inf  LowerLimit=g/2
  Scope{1..6} (6 alike) : Scope
  Sum : Sum  Inputs=|+-
  Sum1 : Sum  Inputs=|+-
  Sum2 : Sum  Inputs=|++
  Sum4 : Sum  Inputs=---
  Trigonometric Function : Trigonometry  Operator=cos
  U3 (m/s^2) : Outport
  wires:
  Gain/1 -> Scope3/1, Sum4/3
  Discrete-Time Integrator/1 -> Gain/1
  K2/1 -> Scope5/1, Sum4/2
  K1/1 -> K3/1
  Sum4/1 -> Sum2/1
  Discrete Derivative1/1 -> IC/1
  Discrete Derivative6/1 -> IC1/1
  z_u/1 -> Discrete Derivative1/1, Mux/1, Sum/1
  Sum/1 -> K1/1, Discrete-Time Integrator/1  "ex"
  Sum1/1 -> K2/1  "ev"
  z_bar/1 -> Mux/2, Sum/2, Discrete Derivative6/1
  Mux/1 -> Scope1/1
  Mux1/1 -> Scope2/1
  Saturation1/1 -> U3 (m/s^2)/1, Scope4/1
  IC/1 -> Mux1/1, Sum1/1
  IC1/1 -> Mux1/2, Sum1/2
  K3/1 -> Scope6/1, Sum4/1
  [theta_u] -> Trigonometric Function/1
  Trigonometric Function/1 -> Divide/2
  Sum2/1 -> Saturation1/1
  Constant/1 -> Divide/1
  Divide/1 -> Sum2/2

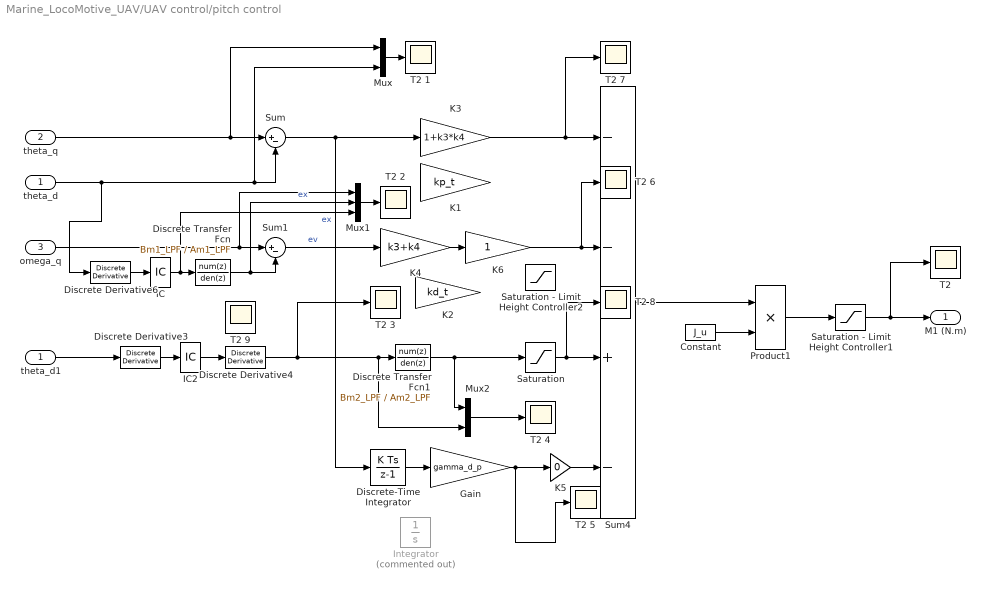
== system Marine_LocoMotive_UAV/UAV control/pitch control ==
  theta_d : Inport
  theta_q : Inport  Port=2
  omega_q : Inport  Port=3
  Constant : Constant  Value=J_u
  Discrete Transfer Fcn : DiscreteTransferFcn  Numerator=Bm1_LPF  Denominator=Am1_LPF
  Discrete Transfer Fcn1 : DiscreteTransferFcn  Numerator=Bm2_LPF  Denominator=Am2_LPF
  Discrete Derivative3 : simulink/Discrete/Discrete Derivative  gainval=1.0  ICPrevScaledInput=Theta0/T  OutMin=[]  OutMax=[]  OutDataType=fixdt(1, 16)  OutScaling=2^-10  DoSatur=off
  Discrete Derivative4 : simulink/Discrete/Discrete Derivative  gainval=1.0  ICPrevScaledInput=0.0  OutMin=[]  OutMax=[]  OutDataType=fixdt(1, 16)  OutScaling=2^-10  DoSatur=off
  Discrete Derivative6 : simulink/Discrete/Discrete Derivative  gainval=1.0  ICPrevScaledInput=Theta0/T  OutMin=[]  OutMax=[]  OutDataType=fixdt(1, 16)  OutScaling=2^-10  DoSatur=off
  Discrete-Time Integrator : DiscreteIntegrator  SampleTime=-1  LimitOutput=on  UpperSaturationLimit=dc_M_p  LowerSaturationLimit=-dc_M_p  ICPrevOutput=DiscIntNeverNeededParam  ICPrevScaledInput=DiscIntNeverNeededParam
  Gain : Gain  Gain=gamma_d_p
  IC : InitialCondition  Value=0
  IC2 : InitialCondition  Value=0
  Integrator : Integrator  Commented=on  LimitOutput=on  UpperSaturationLimit=dc_M_p  LowerSaturationLimit=-dc_M_p
  K1 : Gain  Gain=kp_t
  K2 : Gain  Gain=kd_t
  K3 : Gain  Gain=1+k3*k4
  K4 : Gain  Gain=k3+k4
  K5 : Gain  Gain=0
  K6 : Gain
  Mux : Mux  Inputs=2
  Mux1 : Mux  Inputs=3
  Mux2 : Mux  Inputs=2
  Product1 : Product
  Saturation : Saturate  UpperLimit=[5]  LowerLimit=[-5]
  Saturation - Limit Height Controller1 : Saturate  UpperLimit=0.8  LowerLimit=-0.8
  Saturation - Limit Height Controller2 : Saturate  UpperLimit=15  LowerLimit=-15
  Sum : Sum  Inputs=|+-
  Sum1 : Sum  Inputs=|+-
  Sum4 : Sum  Inputs=--+-
  T2 {,1..9} (10 alike) : Scope
  theta_d1 : InportShadow
  M1 (N.m) : Outport
  wires:
  Product1/1 -> Saturation - Limit Height Controller1/1
  Saturation - Limit Height Controller1/1 -> "T2 "/1, M1 (N.m)/1
  Sum1/1 -> K4/1  "ev"
  Sum4/1 -> Product1/1
  Discrete Derivative6/1 -> IC/1
  Discrete Derivative3/1 -> IC2/1
  Discrete Transfer Fcn1/1 -> Mux2/1, Saturation/1
  Sum/1 -> K3/1, Discrete-Time Integrator/1  "ex"
  K3/1 -> T2 7/1, Sum4/1
  K4/1 -> K6/1
  Discrete-Time Integrator/1 -> Gain/1
  Gain/1 -> K5/1, T2 5/1
  Constant/1 -> Product1/2
  Mux/1 -> T2 1/1
  theta_q/1 -> Mux/1, Sum/1
  omega_q/1 -> Mux1/1, Sum1/1
  Mux1/1 -> T2 2/1
  Discrete Transfer Fcn/1 -> Mux1/2, Sum1/2  "ex"
  Discrete Derivative4/1 -> Mux2/2, Discrete Transfer Fcn1/1, T2 3/1
  theta_d/1 -> Mux/2, Sum/2, Discrete Derivative6/1
  Saturation/1 -> T2 8/1, Sum4/3
  IC/1 -> Mux1/3, Discrete Transfer Fcn/1
  theta_d1/1 -> Discrete Derivative3/1
  IC2/1 -> Discrete Derivative4/1
  K5/1 -> Sum4/4
  Mux2/1 -> T2 4/1
  K6/1 -> T2 6/1, Sum4/2

== system Marine_LocoMotive_UAV/UAV control/u_T ==
  note: PID
  alpha : Inport
  T_bar : Inport  Port=2
  V_bar : Inport  Port=3
  Xb_dot : Inport  Port=4
  Xb_ddot : Inport  Port=5
  Add1 : Sum  Inputs=+++
  Add2 : Sum  Inputs=+++
  Add3 : Sum
  Discrete Derivative1 : simulink/Discrete/Discrete Derivative  gainval=1.0  ICPrevScaledInput=V_bar/T  OutMin=[]  OutMax=[]  OutDataType=fixdt(1, 16)  OutScaling=2^-10  DoSatur=off
  Discrete-Time Integrator1 : DiscreteIntegrator  SampleTime=-1  LimitOutput=on  UpperSaturationLimit=10  LowerSaturationLimit=-10  ICPrevOutput=DiscIntNeverNeededParam  ICPrevScaledInput=DiscIntNeverNeededParam
  Gain1 : Gain  Gain=kd_T
  Gain11 : Gain  Gain=ki_T
  Gain14 : Gain
  Gain2 : Gain  Gain=kp_T
  Gain3 : Gain  Gain=m_u*g
  Gain5 : Gain  Gain=m_u+1.05*m_b
  IC1 : InitialCondition  Value=0
  Product : Product
  Saturation1 : Saturate  UpperLimit=inf  LowerLimit=0
  Scope{1..7,20} (8 alike) : Scope
  Sum5 : Sum  Inputs=|+-
  Sum6 : Sum  Inputs=|+-
  Trigonometric Function : Trigonometry
  V_bar1 : InportShadow  Port=3
  xb_ddot : Selector  InputPortWidth=2  IndexOptions=Index vector (dialog)  Indices=1  OutputSizes=1
  xb_dot : Selector  InputPortWidth=2  IndexOptions=Index vector (dialog)  Indices=1  OutputSizes=1
  u_T : Outport
  wires:
  Product/1 -> Scope7/1, Add2/3
  Discrete-Time Integrator1/1 -> Scope5/1, Add1/2
  Sum6/1 -> Gain1/1
  Gain3/1 -> Add3/1, Add2/1
  Sum5/1 -> Scope4/1, Gain11/1, Gain2/1
  Add1/1 -> Gain5/1
  Gain2/1 -> Scope6/1, Add1/1
  V_bar/1 -> Discrete Derivative1/1, Sum5/1
  T_bar/1 -> Add3/2, Add2/2
  alpha/1 -> Trigonometric Function/1
  xb_dot/1 -> Sum5/2
  Gain1/1 -> Add1/3, Scope20/1
  Trigonometric Function/1 -> Gain3/1
  Discrete Derivative1/1 -> IC1/1
  Gain11/1 -> Discrete-Time Integrator1/1
  Gain14/1 -> Sum6/2
  xb_ddot/1 -> Scope3/1, Gain14/1
  Xb_ddot/1 -> xb_ddot/1
  IC1/1 -> Sum6/1
  Xb_dot/1 -> xb_dot/1
  Add2/1 -> Scope1/1, Saturation1/1  "u_T"
  Saturation1/1 -> u_T/1
  Add3/1 -> Scope2/1
  Gain5/1 -> Product/1
  V_bar1/1 -> Product/2

== system Marine_LocoMotive_UAV/UAV control/u_T1 ==
  note: PID
  alpha : Inport
  T_bar : Inport  Port=2
  V_bar : Inport  Port=3
  Xb_dot : Inport  Port=4
  Xb_ddot : Inport  Port=5
  Add1 : Sum  Inputs=+++
  Add2 : Sum  Inputs=+++
  Add3 : Sum
  Discrete Derivative1 : simulink/Discrete/Discrete Derivative  gainval=1.0  ICPrevScaledInput=V_bar/T  OutMin=[]  OutMax=[]  OutDataType=fixdt(1, 16)  OutScaling=2^-10  DoSatur=off
  Discrete-Time Integrator1 : DiscreteIntegrator  SampleTime=-1  LimitOutput=on  UpperSaturationLimit=10  LowerSaturationLimit=-10  ICPrevOutput=DiscIntNeverNeededParam  ICPrevScaledInput=DiscIntNeverNeededParam
  Gain1 : Gain  Gain=kd_T
  Gain11 : Gain  Gain=ki_T/2*4
  Gain14 : Gain  Gain=0
  Gain2 : Gain  Gain=kp_T*2*4
  Gain3 : Gain  Gain=m_u*g
  Gain5 : Gain  Gain=m_u
  Gain7 : Gain
  IC1 : InitialCondition  Value=0
  Saturation1 : Saturate  UpperLimit=inf  LowerLimit=0
  Scope{1..3,5..7,9,19..20,23} (10 alike) : Scope
  Sum5 : Sum  Inputs=|+-
  Sum6 : Sum  Inputs=|+-
  Trigonometric Function : Trigonometry
  xb_ddot : Selector  InputPortWidth=2  IndexOptions=Index vector (dialog)  Indices=1  OutputSizes=1
  xb_dot : Selector  InputPortWidth=2  IndexOptions=Index vector (dialog)  Indices=1  OutputSizes=1
  u_T : Outport
  wires:
  Add3/1 -> Scope2/1
  Saturation1/1 -> u_T/1
  Add2/1 -> Saturation1/1, Scope1/1  "u_T"
  Xb_dot/1 -> xb_dot/1
  IC1/1 -> Sum6/1
  Xb_ddot/1 -> xb_ddot/1, Scope9/1
  xb_ddot/1 -> Gain14/1
  Gain14/1 -> Sum6/2, Scope3/1
  Gain11/1 -> Discrete-Time Integrator1/1
  Gain1/1 -> Gain7/1
  Discrete Derivative1/1 -> IC1/1
  Trigonometric Function/1 -> Gain3/1
  Gain7/1 -> Scope20/1, Add1/3
  xb_dot/1 -> Sum5/2
  alpha/1 -> Trigonometric Function/1
  T_bar/1 -> Scope6/1, Add2/2, Add3/2
  V_bar/1 -> Sum5/1, Discrete Derivative1/1
  Gain2/1 -> Add1/1
  Add1/1 -> Gain5/1
  Sum5/1 -> Gain2/1, Scope19/1, Gain11/1
  Gain3/1 -> Add2/1, Scope5/1, Add3/1
  Sum6/1 -> Gain1/1
  Discrete-Time Integrator1/1 -> Add1/2, Scope23/1
  Gain5/1 -> Scope7/1, Add2/3

== system Marine_LocoMotive_UAV/UAV control/u_T_Lyapunov ==
  note: PID
  alpha : Inport
  T_bar : Inport  Port=2
  V_bar : Inport  Port=3
  Xb_dot : Inport  Port=4
  Xb_ddot : Inport  Port=5
  alphadot : Inport  Port=6
  Add1 : Sum
  Add2 : Sum  Inputs=-++-
  Add4 : Sum  Inputs=+--
  Discrete Derivative1 : simulink/Discrete/Discrete Derivative  gainval=1.0  ICPrevScaledInput=V_bar/T  OutMin=[]  OutMax=[]  OutDataType=fixdt(1, 16)  OutScaling=2^-10  DoSatur=off
  Discrete-Time Integrator1 : DiscreteIntegrator  SampleTime=-1  LimitOutput=on  UpperSaturationLimit=10  LowerSaturationLimit=-10  ICPrevOutput=DiscIntNeverNeededParam  ICPrevScaledInput=DiscIntNeverNeededParam
  Gain11 : Gain  Gain=ki_T*12
  Gain2 : Gain  Gain=kp_T*12
  Gain3 : Gain  Gain=g
  Gain4 : Gain  Gain=Lc_0
  Gain5 : Gain  Gain=m_u
  Gain6 : Gain  Gain=m_u
  IC1 : InitialCondition  Value=0
  Math Function : Math  Operator=square  SaturateOnIntegerOverflow=on
  Product{,1..3} (4 alike) : Product
  Saturation1 : Saturate  UpperLimit=inf  LowerLimit=0
  Scope{1..8} (8 alike) : Scope
  Sum5 : Sum  Inputs=|+-
  Trigonometric Function : Trigonometry
  Trigonometric Function1 : Trigonometry  Operator=cos
  V_bar1 : InportShadow  Port=3
  alpha1 : InportShadow
  tuner : Gain
  xb_dot : Selector  InputPortWidth=2  IndexOptions=Index vector (dialog)  Indices=1  OutputSizes=1
  zb_dot1 : Selector  InputPortWidth=2  IndexOptions=Index vector (dialog)  Indices=2  OutputSizes=1
  u_T : Outport
  wires:
  Trigonometric Function1/1 -> Product/2, Product2/2
  Gain5/1 -> Product/1
  Saturation1/1 -> u_T/1
  Add2/1 -> Scope1/1, Saturation1/1  "u_T"
  Xb_dot/1 -> xb_dot/1
  Gain11/1 -> Discrete-Time Integrator1/1
  Discrete Derivative1/1 -> IC1/1
  Trigonometric Function/1 -> Product1/2, Gain3/1
  xb_dot/1 -> Sum5/1
  alpha/1 -> Trigonometric Function/1
  T_bar/1 -> Scope3/1, Add2/2
  V_bar/1 -> Sum5/2, Discrete Derivative1/1
  Gain2/1 -> Add1/1, Scope6/1
  Add1/1 -> Gain5/1
  Sum5/1 -> Gain2/1, Gain11/1, Scope4/1
  Discrete-Time Integrator1/1 -> Add1/2, Scope5/1
  Product/1 -> tuner/1
  alpha1/1 -> Trigonometric Function1/1
  Xb_ddot/1 -> zb_dot1/1
  zb_dot1/1 -> Product1/1
  alphadot/1 -> Math Function/1
  Math Function/1 -> Gain4/1
  Add4/1 -> Gain6/1
  Gain3/1 -> Add4/3
  Product1/1 -> Add4/2
  Gain4/1 -> Add4/1
  Gain6/1 -> Scope2/1, Add2/1
  IC1/1 -> Scope8/1, Product2/1
  Product2/1 -> Add2/3
  Product3/1 -> Add2/4, Scope7/1
  V_bar1/1 -> Product3/2
  tuner/1 -> Product3/1

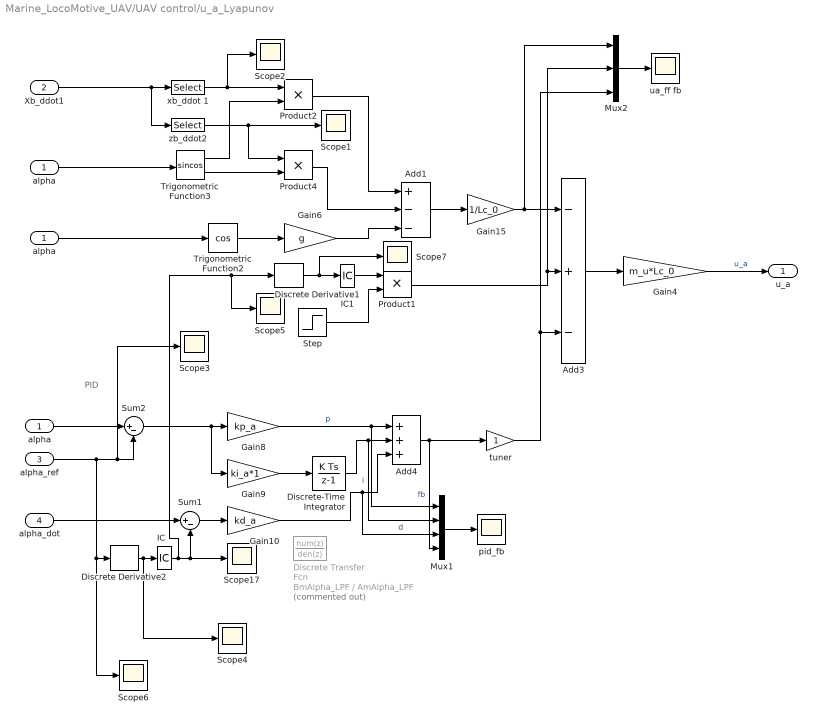
== system Marine_LocoMotive_UAV/UAV control/u_a_Lyapunov ==
  note: PID
  alpha : Inport
  Xb_ddot1 : Inport  Port=2
  alpha_ref : Inport  Port=3
  "alpha_dot " : Inport  Port=4
  " alpha" : InportShadow
  Add1 : Sum  Inputs=+--
  Add3 : Sum  Inputs=-+-
  Add4 : Sum  Inputs=3
  Discrete Transfer Fcn : DiscreteTransferFcn  Commented=on  Numerator=BmAlpha_LPF  Denominator=AmAlpha_LPF
  Discrete Derivative1 : simulink/Discrete/Discrete Derivative  gainval=1.0  ICPrevScaledInput=alpha_bar  OutMin=[]  OutMax=[]  OutDataType=fixdt(1, 16)  OutScaling=2^-10  DoSatur=off
  Discrete Derivative2 : simulink/Discrete/Discrete Derivative  gainval=1.0  ICPrevScaledInput=alpha_bar/T  OutMin=[]  OutMax=[]  OutDataType=fixdt(1, 16)  OutScaling=2^-10  DoSatur=off
  Discrete-Time Integrator : DiscreteIntegrator  SampleTime=-1  LimitOutput=on  UpperSaturationLimit=1  LowerSaturationLimit=-1  ICPrevOutput=DiscIntNeverNeededParam  ICPrevScaledInput=DiscIntNeverNeededParam
  Gain10 : Gain  Gain=kd_a
  Gain15 : Gain  Gain=1/Lc_0
  Gain4 : Gain  Gain=m_u*Lc_0
  Gain6 : Gain  Gain=g
  Gain8 : Gain  Gain=kp_a
  Gain9 : Gain  Gain=ki_a*1
  IC : InitialCondition  Value=0
  IC1 : InitialCondition  Value=0
  Mux1 : Mux
  Mux2 : Mux  Inputs=3
  Product1 : Product
  Product2 : Product
  Product4 : Product
  Scope{1..7,17} (8 alike) : Scope
  Step : Step  Time=250*T  SampleTime=0
  Sum1 : Sum  Inputs=|+-
  Sum2 : Sum  Inputs=|+-
  Trigonometric Function2 : Trigonometry  Operator=cos
  Trigonometric Function3 : Trigonometry  Operator=sincos
  "alpha " : InportShadow
  pid_fb : Scope
  tuner : Gain
  ua_ff fb : Scope
  xb_ddot 1 : Selector  InputPortWidth=2  IndexOptions=Index vector (dialog)  Indices=1  OutputSizes=1
  zb_ddot2 : Selector  InputPortWidth=2  IndexOptions=Index vector (dialog)  Indices=2  OutputSizes=1
  u_a : Outport
  wires:
  Mux2/1 -> ua_ff fb/1
  Gain15/1 -> Mux2/1, Add3/1
  Mux1/1 -> pid_fb/1
  alpha/1 -> Trigonometric Function2/1
  "alpha "/1 -> Trigonometric Function3/1
  " alpha"/1 -> Sum2/1
  Trigonometric Function3/2 -> Product4/2
  Discrete-Time Integrator/1 -> Add4/2, Mux1/2  "i"
  Add1/1 -> Gain15/1
  Trigonometric Function2/1 -> Gain6/1
  Trigonometric Function3/1 -> Product2/2
  Product2/1 -> Add1/1
  Gain9/1 -> Discrete-Time Integrator/1
  xb_ddot 1/1 -> Product2/1, Scope2/1
  Gain10/1 -> Add4/3, Mux1/3  "d"
  Xb_ddot1/1 -> xb_ddot 1/1, zb_ddot2/1
  Add3/1 -> Gain4/1
  Gain8/1 -> Add4/1, Mux1/1  "p"
  zb_ddot2/1 -> Product4/1, Scope1/1
  tuner/1 -> Mux2/3, Add3/3
  Gain4/1 -> u_a/1  "u_a"
  "alpha_dot "/1 -> Sum1/1
  Add4/1 -> tuner/1, Mux1/4  "fb"
  Sum1/1 -> Gain10/1
  Sum2/1 -> Gain8/1, Gain9/1
  Discrete Derivative2/1 -> Scope4/1, IC/1
  Gain6/1 -> Add1/3
  Product4/1 -> Add1/2
  Discrete Derivative1/1 -> Scope7/1, IC1/1
  Product1/1 -> Mux2/2, Add3/2
  alpha_ref/1 -> Scope6/1, Discrete Derivative2/1, Scope3/1, Sum2/2
  IC1/1 -> Product1/1
  Step/1 -> Product1/2
  IC/1 -> Scope5/1, Discrete Derivative1/1, Sum1/2, Scope17/1

== system Marine_LocoMotive_UAV/UAV control/u_alpha ==
  note: PID
  alpha : Inport
  Xb_ddot1 : Inport  Port=2
  alpha_ref : Inport  Port=3
  "alpha_dot " : Inport  Port=4
  " alpha" : InportShadow
  Add3 : Sum  Inputs=+--
  Add4 : Sum  Inputs=3
  Discrete Transfer Fcn : DiscreteTransferFcn  Commented=on  Numerator=BmAlpha_LPF  Denominator=AmAlpha_LPF
  Discrete Derivative2 : simulink/Discrete/Discrete Derivative  gainval=1.0  ICPrevScaledInput=alpha_bar/T  OutMin=[]  OutMax=[]  OutDataType=fixdt(1, 16)  OutScaling=2^-10  DoSatur=off
  Discrete-Time Integrator : DiscreteIntegrator  SampleTime=-1  LimitOutput=on  UpperSaturationLimit=1  LowerSaturationLimit=-1  ICPrevOutput=DiscIntNeverNeededParam  ICPrevScaledInput=DiscIntNeverNeededParam
  Gain10 : Gain  Gain=kd_a
  Gain12 : Gain  Gain=Lc_0
  Gain4 : Gain  Gain=m_u
  Gain6 : Gain  Gain=g
  Gain8 : Gain  Gain=kp_a
  Gain9 : Gain  Gain=ki_a*1
  IC : InitialCondition  Value=0
  Mux1 : Mux
  Mux2 : Mux  Inputs=3
  Product2 : Product
  Product4 : Product
  Scope1 : Scope
  Scope17 : Scope
  Scope2 : Scope
  Sum1 : Sum  Inputs=|+-
  Sum2 : Sum  Inputs=|+-
  Sum7 : Sum  Inputs=|+-
  Trigonometric Function2 : Trigonometry  Operator=cos
  Trigonometric Function3 : Trigonometry  Operator=sincos
  "alpha " : InportShadow
  pid_fb : Scope
  tuner : Gain
  "tuner " : Gain
  ua_ff fb : Scope
  xb_ddot 1 : Selector  InputPortWidth=2  IndexOptions=Index vector (dialog)  Indices=1  OutputSizes=1
  zb_ddot2 : Selector  InputPortWidth=2  IndexOptions=Index vector (dialog)  Indices=2  OutputSizes=1
  u_a : Outport
  wires:
  IC/1 -> Scope17/1, Sum1/2
  Gain6/1 -> Mux2/1, Add3/1
  Sum2/1 -> Gain9/1, Gain8/1
  Sum1/1 -> Gain10/1
  alpha_ref/1 -> Sum2/2, Discrete Derivative2/1
  Add4/1 -> Mux1/4, Gain12/1  "fb"
  "alpha_dot "/1 -> Sum1/1
  Gain4/1 -> u_a/1  "u_a"
  tuner/1 -> Add3/3, Mux2/3
  Product4/1 -> Sum7/2
  zb_ddot2/1 -> Product4/1, Scope1/1
  Gain8/1 -> Mux1/1, Add4/1  "p"
  Add3/1 -> Gain4/1
  Discrete Derivative2/1 -> IC/1
  Xb_ddot1/1 -> zb_ddot2/1, xb_ddot 1/1
  Gain10/1 -> Mux1/3, Add4/3  "d"
  xb_ddot 1/1 -> Scope2/1, Product2/1
  Gain9/1 -> Discrete-Time Integrator/1
  Product2/1 -> Sum7/1
  Trigonometric Function3/1 -> Product2/2
  Trigonometric Function2/1 -> Gain6/1
  Sum7/1 -> "tuner "/1
  Discrete-Time Integrator/1 -> Mux1/2, Add4/2  "i"
  Trigonometric Function3/2 -> Product4/2
  " alpha"/1 -> Sum2/1
  "alpha "/1 -> Trigonometric Function3/1
  alpha/1 -> Trigonometric Function2/1
  Mux1/1 -> pid_fb/1
  "tuner "/1 -> Add3/2, Mux2/2
  Gain12/1 -> tuner/1
  Mux2/1 -> ua_ff fb/1
